simulink model "Q3_W1"  (R2020b)
settings: Solver=VariableStepAuto  StartTime=0.0  StopTime=10.0  MaxStep=0.00002  RelTol=1e-3
settings Model: Creator=hp  LastModifiedBy=hp

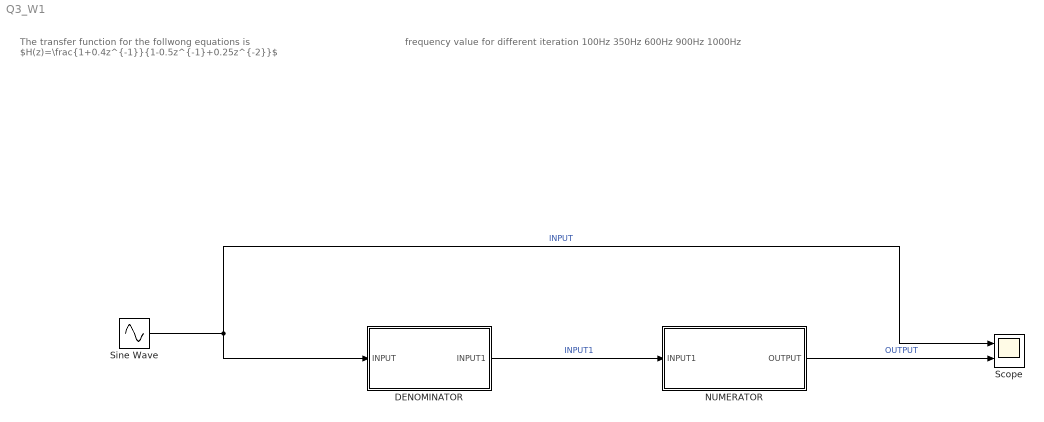
== system Q3_W1 ==
  note: frequency value for different iteration
      | 100Hz
      | 350Hz
      | 600Hz
      | 900Hz
      | 1000Hz
  note: The transfer function for the follwong equations is
      | $H(z)=\frac{1+0.4z^{-1}}{1-0.5z^{-1}+0.25z^{-2}}$
  DENOMINATOR : Subsystem  TreatAsAtomicUnit=on
  NUMERATOR : Subsystem  TreatAsAtomicUnit=on
  Scope : Scope  NumInputPorts=2
  Sine Wave : Sin  Frequency=2*pi*100  SampleTime=0
  wires:
  Sine Wave/1 -> DENOMINATOR/1(INPUT), Scope/1  "INPUT"
  DENOMINATOR/1(INPUT1) -> NUMERATOR/1(INPUT1)  "INPUT1"
  NUMERATOR/1(OUTPUT) -> Scope/2  "OUTPUT"

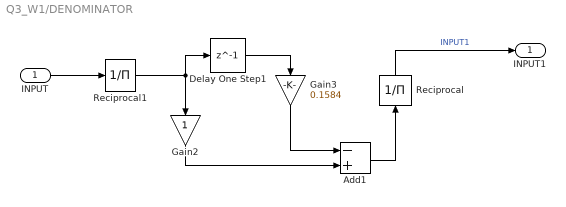
== system Q3_W1/DENOMINATOR ==
  INPUT : Inport
  Add1 : Sum  Inputs=-+
  Delay One Step1 : Delay  DelayLength=1
  Gain2 : Gain
  Gain3 : Gain  Gain=0.1584
  Reciprocal : Product  Inputs=/
  Reciprocal1 : Product  Inputs=/
  INPUT1 : Outport
  wires:
  Add1/1 -> Reciprocal/1
  Reciprocal/1 -> INPUT1/1  "INPUT1"
  Delay One Step1/1 -> Gain3/1
  Reciprocal1/1 -> Delay One Step1/1, Gain2/1
  Gain2/1 -> Add1/2
  Gain3/1 -> Add1/1
  INPUT/1 -> Reciprocal1/1

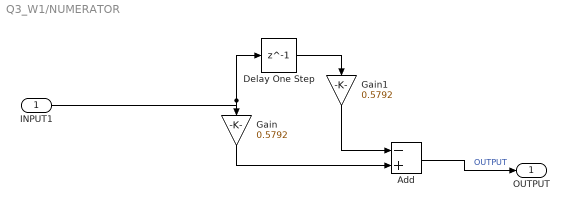
== system Q3_W1/NUMERATOR ==
  INPUT1 : Inport
  Add : Sum  Inputs=-+
  Delay One Step : Delay  DelayLength=1
  Gain : Gain  Gain=0.5792
  Gain1 : Gain  Gain=0.5792
  OUTPUT : Outport
  wires:
  Gain1/1 -> Add/1
  Gain/1 -> Add/2
  INPUT1/1 -> Delay One Step/1, Gain/1
  Delay One Step/1 -> Gain1/1
  Add/1 -> OUTPUT/1  "OUTPUT"
